simulink model "CircuitoRC"  (R2020b)
settings: Solver=ode45  StartTime=0.0  StopTime=10.0  FixedStep=0.01  MaxStep=0.1  RelTol=1e-3
values from neighbouring files (symbols this model uses):
  C = R*C0    [tri_plot.m]
  R = [cos(theta) -sin(theta) tx ... (first row only)    [tri_plot.m]
settings Model: Creator=Stefano  LastModifiedBy=Stefano

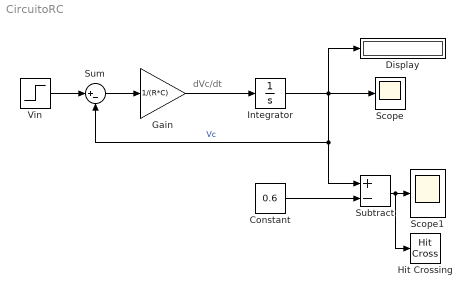
== system CircuitoRC ==
  note: dVc/dt
  Constant : Constant  Value=0.6
  Display : Display
  Gain : Gain  Gain=1/(R*C)
  Hit Crossing : HitCross
  Integrator : Integrator
  Scope : Scope
  Scope1 : Scope
  Subtract : Sum  Inputs=+-
  Sum : Sum  Inputs=|+-
  Vin : Step  Time=2  SampleTime=0
  wires:
  Gain/1 -> Integrator/1
  Integrator/1 -> Scope/1, Display/1, Subtract/1, Sum/2  "Vc"
  Sum/1 -> Gain/1
  Vin/1 -> Sum/1
  Constant/1 -> Subtract/2
  Subtract/1 -> Hit Crossing/1, Scope1/1
